simulink model "oxidationNMPC"  (R2023a)
settings: Solver=VariableStepAuto  StartTime=0.0  StopTime=Tstop  RelTol=1e-3
values from neighbouring files (symbols this model uses):
  PredictionHorizon = 10    [NonlinearAndGSMPCControlOfAnEthyleneOxidationPlant1.m]
  Ts = 5    [NonlinearAndGSMPCControlOfAnEthyleneOxidationPlant1.m]
  uLow = [0.38 0.5]    [NonlinearAndGSMPCControlOfAnEthyleneOxidationPlant1.m]
  xLow = fsolve(@(x) oxidationStateFcn(x,uLow),[1 0.3 0.03 1],options)    [NonlinearAndGSMPCControlOfAnEthyleneOxidationPlant1.m]
undefined symbols (not defined in the file or in its folder): ref
libraries: mpclib x1
settings Model: Creator=The MathWorks, Inc.  LastModifiedBy=The MathWorks, Inc.
settings SolverCC: AlgebraicLoopSolver=TrustRegion
settings DataIOCC: SaveFormat=Array  SaveOutput=off  SignalLogging=off  DSMLogging=off  SaveTime=off  ReturnWorkspaceOutputs=off
settings DebuggingCC: UnconnectedInputMsg=warning  UnconnectedOutputMsg=warning  UnconnectedLineMsg=warning  ArithmeticOperatorsInVariantConditions=warning
settings ModelReferenceCC: EnableRefExpFcnMdlSchedulingChecks=on
settings SFSimCC: SimUseLocalCustomCode=off  CustomCodeUndefinedFunction=UseInterfaceOnly
settings RTWCC: RTWUseLocalCustomCode=off
settings CodeAppCC: StateflowObjectComments=on
settings GRTTargetCC: TargetLangStandard=C89/C90 (ANSI)
settings ConfigComp: CovMetricSettings=dsw  CovSaveCumulativeToWorkspaceVar=on  CovSaveSingleToWorkspaceVar=on  CovExternalEMLEnable=off

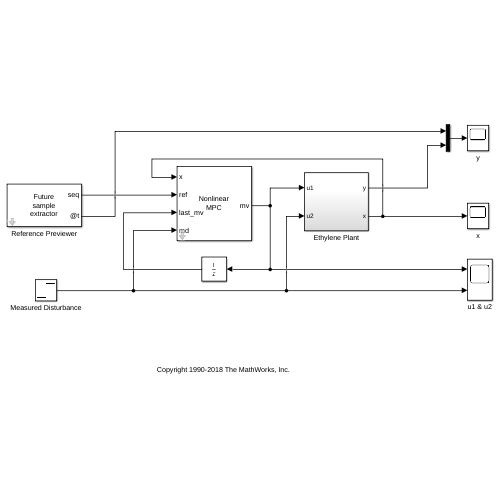
[thumbnail: Simulink's stored preview of the top-level diagram]
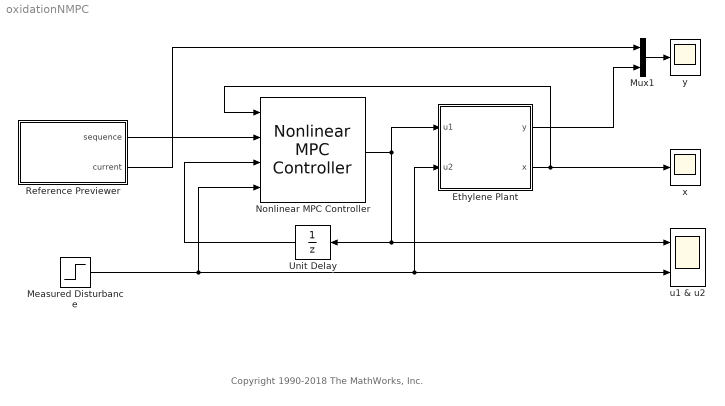
== system oxidationNMPC ==
  note: Copyright 1990-2018 The MathWorks, Inc.
  Ethylene Plant : Subsystem
  Measured Disturbance : Step  Time=200  Before=uLow(2)  After=uLow(2)+0.1  SampleTime=Ts
  Mux1 : Mux  Inputs=2
  Nonlinear MPC Controller : mpclib/Nonlinear MPC Controller  SCDEnableBlockLinearizationSpecification=on  nlmpcobj=nlobj  UseObjectTs=on  UseMEX=off  md_enabled=on  mvtarget_enabled=off  param_enabled=off  cost_enabled=off  mvseq_enabled=off  stateseq_enabled=off  ovseq_enabled=off  slack_enabled=off  status_enabled=off  ov_min=off  ov_max=off  mv_min=off  mv_max=off  mvrate_min=off  mvrate_max=off  state_min=off  state_max=off  ov_weight=off  mv_weight=off  mvrate_weight=off  ecr_weight=off  nlp_initialize=off
  Reference Previewer : Subsystem  mask{signal=ref, ts=Ts, steps=PredictionHorizon}
      mask prompts: signal "Signal name"; ts "Sampling time"; steps "Number of previewing steps"
      mask init:
      | ts = evalin('base',get_param(gcbh,'ts'));
      | signal = evalin('base',get_param(gcbh,'signal'));
      | steps = evalin('base',get_param(gcbh,'steps'));
      | data = mpc_previewer_maskinit(signal,ts);
      mask Display:
      | fprintf('Future\nsample\nextractor');
      | port_label('output', 1, 'seq')
      | port_label('output', 2, '@t')
  Unit Delay : UnitDelay  InitialCondition=uLow(1)  SampleTime=-1  HasFrameUpgradeWarning=on
  u1 & u2 : Scope  NumInputPorts=2
  x : Scope
  y : Scope
  wires:
  Nonlinear MPC Controller/1 -> Ethylene Plant/1(u1), Unit Delay/1, u1 & u2/1
  Mux1/1 -> y/1
  Reference Previewer/2(current) -> Mux1/1
  Ethylene Plant/2(x) -> Nonlinear MPC Controller/1, x/1
  Reference Previewer/1(sequence) -> Nonlinear MPC Controller/2
  Measured Disturbance/1 -> Nonlinear MPC Controller/4, Ethylene Plant/2(u2), u1 & u2/2
  Ethylene Plant/1(y) -> Mux1/2
  Unit Delay/1 -> Nonlinear MPC Controller/3

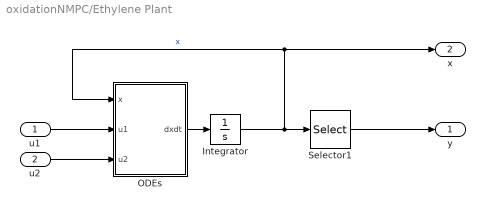
== system oxidationNMPC/Ethylene Plant ==
  u1 : Inport
  u2 : Inport  Port=2
  Integrator : Integrator  InitialCondition=xLow
  ODEs : MATLAB Function  TreatAsAtomicUnit=on
  Selector1 : Selector  InputPortWidth=4  IndexOptions=Index vector (dialog)  Indices=3  OutputSizes=1
  y : Outport  VectorParamsAs1DForOutWhenUnconnected=off
  x : Outport  Port=2  VectorParamsAs1DForOutWhenUnconnected=off
  wires:
  u2/1 -> ODEs/3(u2)
  u1/1 -> ODEs/2(u1)
  Selector1/1 -> y/1
  ODEs/1(dxdt) -> Integrator/1
  Integrator/1 -> x/1, ODEs/1(x), Selector1/1  "x"

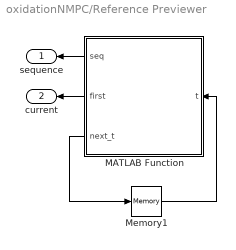
== system oxidationNMPC/Reference Previewer ==
  MATLAB Function : MATLAB Function  TreatAsAtomicUnit=on
  Memory1 : Memory  InheritSampleTime=on  LinearizeAsDelay=on
  sequence : Outport  VectorParamsAs1DForOutWhenUnconnected=off
  current : Outport  Port=2  VectorParamsAs1DForOutWhenUnconnected=off
  wires:
  MATLAB Function/3(next_t) -> Memory1/1
  Memory1/1 -> MATLAB Function/1(t)
  MATLAB Function/2(first) -> current/1
  MATLAB Function/1(seq) -> sequence/1

== matlab function oxidationNMPC/Ethylene Plant/ODEs ==
  data: dxdt output; x input; u1 input; u2 input
function dxdt = fcn(x, u1, u2)

% Compute time derivatives and outputs for the ethylene oxide reactor

% Compute state derivatives
dxdt = oxidationStateFcn(x, [u1;u2]);

== matlab function oxidationNMPC/Reference Previewer/MATLAB Function ==
  settings: updateMethod=DISCRETE  sampleTime=ts
  data: data parameter; seq output; steps parameter; t input; first output; next_t output
function [seq,first,next_t] = fcn(data,steps,t)
%#codegen
[seq,first,next_t] = mpcblock_preview('ref',data,steps,t);
